simulink model "house_heating_system"  (R2018b)
settings: Solver=VariableStepAuto  StartTime=0.0  StopTime=24  RelTol=1e-3
model workspace (MAT data in the model file):
  M_heater_air = 3600
  R_equivalent = 4.329e-07
  T_heater = 50
  T_roomIC = 20
  c_air = 1005.4
  m_room_air = 1470
settings Model: Creator=mikoto  LastModifiedBy=mikoto

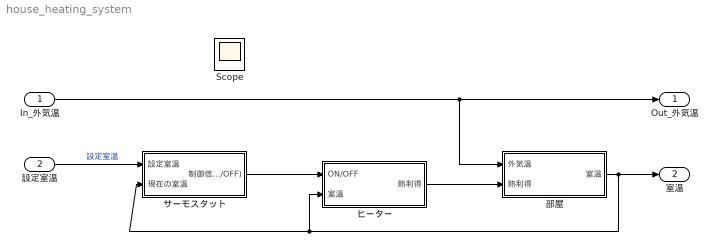
== system house_heating_system ==
  In_外気温 : Inport
  設定室温 : Inport  Port=2
  サーモスタット : Subsystem
  ヒーター : Subsystem
  部屋 : Subsystem
  Out_外気温 : Outport
  室温 : Outport  Port=2
  Scope : Scope
  wires:
  設定室温/1 -> サーモスタット/1(設定室温)  "設定室温"
  サーモスタット/1(制御信号 (ON/OFF)) -> ヒーター/1(ON/OFF)
  ヒーター/1(熱利得) -> 部屋/2(熱利得)
  部屋/1(室温) -> 室温/1, ヒーター/2(室温), サーモスタット/2(現在の室温)
  In_外気温/1 -> 部屋/1(外気温), Out_外気温/1

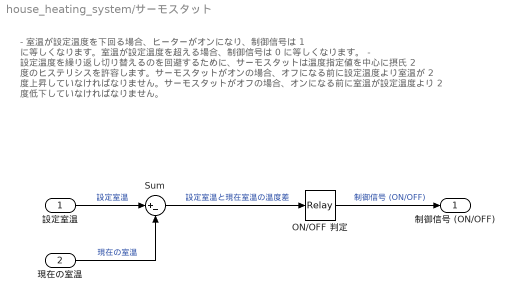
== system house_heating_system/サーモスタット ==
  note: - 室温が設定温度を下回る場合、ヒーターがオンになり、制御信号は 1 に等しくなります。室温が設定温度を超える場合、制御信号は 0 に等しくなります。
      | - 設定温度を繰り返し切り替えるのを回避するために、サーモスタットは温度指定値を中心に摂氏 2 度のヒステリシスを許容します。サーモスタットがオンの場合、オフになる前に設定温度より室温が 2 度上昇していなければなりません。サーモスタットがオフの場合、オンになる前に室温が設定温度より 2 度低下していなければなりません。
  設定室温 : Inport
  現在の室温 : Inport  Port=2
  ON/OFF 判定 : Relay  OnSwitchValue=2  OffSwitchValue=-2
  Sum : Sum  Inputs=|+-
  制御信号 (ON/OFF) : Outport
  wires:
  設定室温/1 -> Sum/1  "設定室温"
  現在の室温/1 -> Sum/2  "現在の室温"
  Sum/1 -> ON/OFF 判定/1  "設定室温と現在室温の温度差"
  ON/OFF 判定/1 -> 制御信号 (ON/OFF)/1  "制御信号 (ON/OFF)"

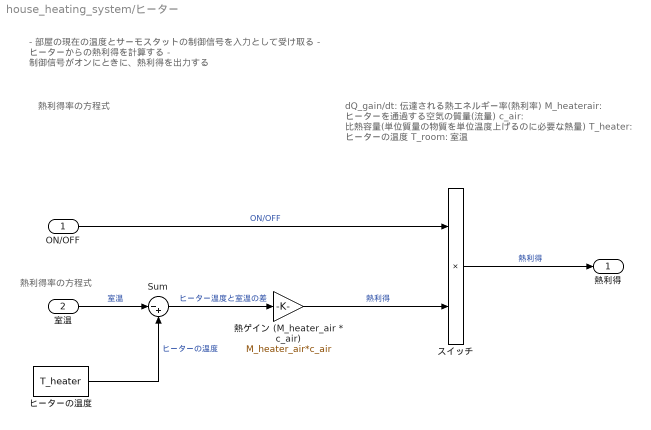
== system house_heating_system/ヒーター ==
  note: - 部屋の現在の温度とサーモスタットの制御信号を入力として受け取る
      | - ヒーターからの熱利得を計算する
      | - 制御信号がオンにときに、熱利得を出力する
  note: 熱利得率の方程式
  note: dQ_gain/dt: 伝達される熱エネルギー率(熱利率)
      | M_heaterair: ヒーターを通過する空気の質量(流量)
      | c_air: 比熱容量(単位質量の物質を単位温度上げるのに必要な熱量)
      | T_heater: ヒーターの温度
      | T_room: 室温
  note: 熱利得率の方程式
  ON/OFF : Inport
  室温 : Inport  Port=2
  Sum : Sum  Inputs=|-+
  スイッチ : Product
  ヒーターの温度 : Constant  Value=T_heater
  熱ゲイン (M_heater_air * c_air) : Gain  Gain=M_heater_air*c_air
  熱利得 : Outport
  wires:
  ON/OFF/1 -> スイッチ/1  "ON/OFF"
  ヒーターの温度/1 -> Sum/2  "ヒーターの温度"
  室温/1 -> Sum/1  "室温"
  Sum/1 -> 熱ゲイン (M_heater_air * c_air)/1  "ヒーター温度と室温の差"
  スイッチ/1 -> 熱利得/1  "熱利得"
  熱ゲイン (M_heater_air * c_air)/1 -> スイッチ/2  "熱利得"

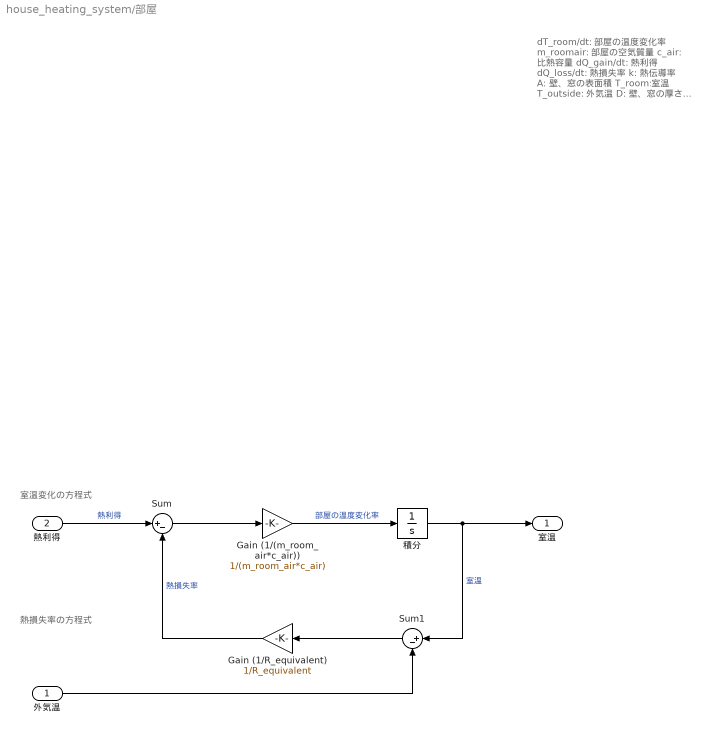
== system house_heating_system/部屋 ==
  note: 熱損失率の方程式
  note: 室温変化の方程式
  note: dT_room/dt: 部屋の温度変化率
      | m_roomair: 部屋の空気質量
      | c_air: 比熱容量
      | dQ_gain/dt: 熱利得
      | dQ_loss/dt: 熱損失率
      |
      | k: 熱伝導率
      | A: 壁、窓の表面積
      | T_room:室温
      | T_outside: 外気温
      | D: 壁、窓の厚さ
      | R: 熱抵抗
  外気温 : Inport
  熱利得 : Inport  Port=2
  Gain (1/(m_room_air*c_air)) : Gain  Gain=1/(m_room_air*c_air)
  Gain (1/R_equivalent) : Gain  Gain=1/R_equivalent
  Sum : Sum  Inputs=|+-
  Sum1 : Sum  Inputs=|+-
  積分 : Integrator  InitialCondition=T_roomIC
  室温 : Outport
  wires:
  熱利得/1 -> Sum/1  "熱利得"
  Gain (1/(m_room_air*c_air))/1 -> 積分/1  "部屋の温度変化率"
  Sum/1 -> Gain (1/(m_room_air*c_air))/1
  Gain (1/R_equivalent)/1 -> Sum/2  "熱損失率"
  積分/1 -> Sum1/1, 室温/1  "室温"
  外気温/1 -> Sum1/2
  Sum1/1 -> Gain (1/R_equivalent)/1
